simulink model "nao_cm"  (R2022b)
settings: Solver=VariableStepAuto  StartTime=0.0  StopTime=200  RelTol=1e-3
undefined symbols (not defined in the file or in its folder): sigbuilder_block, X, Y, Z
libraries: sm_lib x2657, nesl_utility x5
(part 1 of 45)
settings Model: Creator=josep  LastModifiedBy=josep

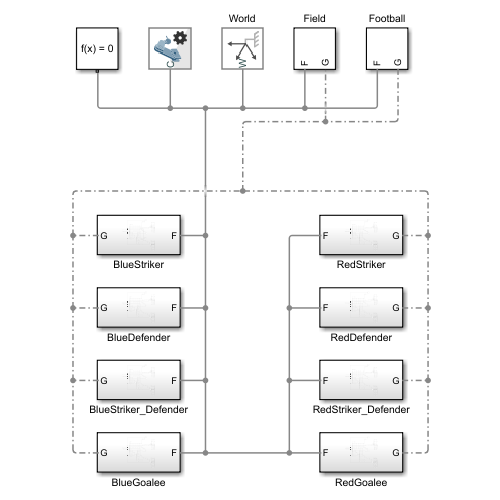
[thumbnail: Simulink's stored preview of the top-level diagram]
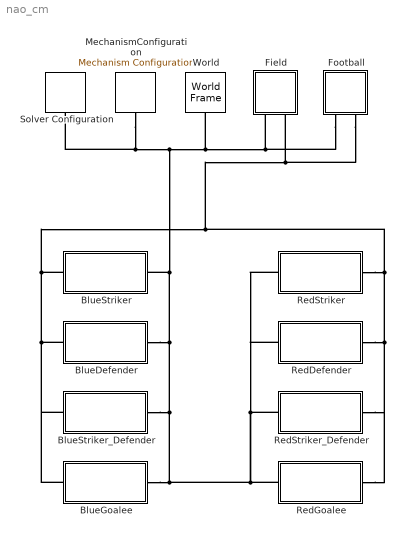
== system nao_cm ==
  BlueDefender : Subsystem
  BlueGoalee : Subsystem
  BlueStriker : Subsystem
  BlueStriker_Defender : Subsystem
  Field : Subsystem
  Football : Subsystem
  MechanismConfiguration : sm_lib/Utilities/Mechanism Configuration  UniformGravity=Constant  GravityVector=[0 0 -9.80665]  GravityUnits=m/s^2  LinearizationDelta=0.001  JointModeTransitionNonlinearIterations=2
  RedDefender : Subsystem
  RedGoalee : Subsystem
  RedStriker : Subsystem
  RedStriker_Defender : Subsystem
  Solver Configuration : nesl_utility/Solver Configuration  PhysicalDomain=network_engine_domain  SubClassName=solver  LeftPortType=input  RightPortType=generic  Tones=[]  Harmonics=[]  SimulateNoise=off  Profile=off  UseLocalSampling=off  EnableSwitchedLinearOptims=on  FrequencyDomain=off  UseCCode=off  RelTol=0.001  AbsTol=0.001  MinStep=1e-09  ToWorkspace=off  RevertToSquareIcSolve=off  NumHomotopyIterations=100  PhasorMode=off  PhasorModeNumHarmonics=1  ConsistencySolver=NEWTON_XTOL_AFTER_FTOL  IndexReductionMethod=DerivativeReplacement  DoDC=off  ResidualTolerance=1e-09  ConsistencyTolSource=GLOBAL  ConsistencyAbsTol=0.001  ConsistencyRelTol=0.001  ConsistencyTolFactor=0.001  UseLocalSolver=off  LocalSolverChoice=NE_BACKWARD_EULER_ADVANCER  ResolveIndetEquations=on  FunctionEvalNumThread=1  LocalSolverSampleTime=0.001  DoFixedCost=off  MaxNonlinIter=3  MaxModeIter=2  ComputeImpulses=off  ImpulseIterations=2  LinearAlgebra=auto  LinearAlgebraNumThread=0  EquationFormulation=NE_TIME_EF  DelaysMemoryBudget=1024  AutomaticFiltering=on  FilteringTimeConstant=0.001  PartitionStorageMethod=AS_NEEDED  PartitionMemoryBudget=1024  PartitionMethod=ROBUST
  World : sm_lib/Frames and Transforms/World Frame
  connections:
  MechanismConfiguration/RConn1 -- Solver Configuration/RConn1 -- Football/LConn1 -- Field/LConn1 -- World/RConn1 -- BlueStriker/LConn1 -- BlueDefender/LConn1 -- RedStriker/LConn1 -- RedDefender/LConn1 -- RedStriker_Defender/LConn1 -- RedGoalee/LConn1 -- BlueGoalee/LConn1 -- BlueStriker_Defender/LConn1
  BlueStriker/RConn1 -- RedGoalee/RConn1 -- RedStriker_Defender/RConn1 -- RedDefender/RConn1 -- RedStriker/RConn1 -- Field/LConn2 -- Football/LConn2 -- BlueDefender/RConn1 -- BlueStriker_Defender/RConn1 -- BlueGoalee/RConn1
